simulink model "Demo_LaneKeeping_cs"  (Simulink 8.7)
settings: Solver=ode5  SolverMode=SingleTasking  StartTime=0.0  StopTime=38  FixedStep=1/20  RelTol=1e-3
model workspace (MAT data in the model file):
  mbox_table.block_array(1).src = 'built-in/Subsystem'
  mbox_table.block_array(1).dest = 'Demo_LaneKeeping_cs/Mazda_RX8_1'
  mbox_table.block_array(1).mode = 0
  mbox_table.block_array(2).src = 'simulink/Sinks/Out1'
  mbox_table.block_array(2).dest = 'Demo_LaneKeeping_cs/Mazda_RX8_1/STATE_Mazda_RX8_1'
  mbox_table.block_array(2).mode = 0
  mbox_table.block_array(3).src = 'PreScanSimulinkLibrary/State'
  mbox_table.block_array(3).dest = 'Demo_LaneKeeping_cs/STATE_Mazda_RX8_1'
  mbox_table.block_array(3).mode = 0
  mbox_table.block_array(4).src = 'PreScanSimulinkLibrary/SELF'
  mbox_table.block_array(4).dest = 'Demo_LaneKeeping_cs/SELF_Mazda_RX8_1'
  mbox_table.block_array(4).mode = 0
  mbox_table.block_array(5).src = 'simulink/Sources/In1'
  mbox_table.block_array(5).dest = 'Demo_LaneKeeping_cs/Mazda_RX8_1/SELF_Mazda_RX8_1'
  mbox_table.block_array(5).mode = 0
  mbox_table.block_array(6).src = 'PreScanSimulinkLibrary/DemuxSELF'
  mbox_table.block_array(6).dest = 'Demo_LaneKeeping_cs/Mazda_RX8_1/SELF_Demux'
  mbox_table.block_array(6).mode = 0
  mbox_table.block_array(7).src = 'PreScanSimulinkLibrary/LaneMarkerSensor'
  mbox_table.block_array(7).dest = 'Demo_LaneKeeping_cs/LaneMarkerSensor_1'
  mbox_table.block_array(7).mode = 0
  mbox_table.block_array(8).src = 'simulink/Sources/In1'
  mbox_table.block_array(8).dest = 'Demo_LaneKeeping_cs/Mazda_RX8_1/LaneMarkerSensor_1'
  mbox_table.block_array(8).mode = 0
  mbox_table.block_array(9).src = 'PreScanSimulinkLibrary/LaneMarkerSensor_Data'
  mbox_table.block_array(9).dest = 'Demo_LaneKeeping_cs/Mazda_RX8_1/LaneMarkerSensor_1_Data'
  mbox_table.block_array(9).mode = 0
  mbox_table.block_array(10).src = 'simulink/Sinks/Out1'
  mbox_table.block_array(10).dest = 'Demo_LaneKeeping_cs/Mazda_RX8_1/VISUWheels_Mazda_RX8_1'
  mbox_table.block_array(10).mode = 0
  mbox_table.block_array(11).src = 'PreScanSimulinkLibrary/VisuWheels'
  mbox_table.block_array(11).dest = 'Demo_LaneKeeping_cs/VISUWheels_Mazda_RX8_1'
  mbox_table.block_array(11).mode = 0
  mbox_table.block_array(12).src = 'PreScanSimulinkLibrary/MuxWheels'
  mbox_table.block_array(12).dest = 'Demo_LaneKeeping_cs/Mazda_RX8_1/VISUWheels_Mux'
  mbox_table.block_array(12).mode = 0
  mbox_table.block_array(13).src = 'simulink/Sinks/Out1'
  mbox_table.block_array(13).dest = 'Demo_LaneKeeping_cs/Mazda_RX8_1/VISUSteer_Mazda_RX8_1'
  mbox_table.block_array(13).mode = 0
  mbox_table.block_array(14).src = 'PreScanSimulinkLibrary/VisuSteer'
  mbox_table.block_array(14).dest = 'Demo_LaneKeeping_cs/VISUSteer_Mazda_RX8_1'
  mbox_table.block_array(14).mode = 0
  mbox_table.block_array(15).src = 'PreScanSimulinkLibrary/MuxSteer'
  mbox_table.block_array(15).dest = 'Demo_LaneKeeping_cs/Mazda_RX8_1/VISUSteer_Mux'
  mbox_table.block_array(15).mode = 0
  mbox_table.block_array(16).src = 'PreScanSimulinkLibrary/Simple_Vehicle_Dynamics'
  mbox_table.block_array(16).dest = 'Demo_LaneKeeping_cs/Mazda_RX8_1/Dynamics_Simple'
  mbox_table.block_array(16).mode = 0
  mbox_table.block_array(17).src = 'simulink/Sources/Constant'
  mbox_table.block_array(17).dest = 'Demo_LaneKeeping_cs/Mazda_RX8_1/Auto_Gear'
  mbox_table.block_array(17).mode = 0
  mbox_table.block_array(18).src = 'SimCoreLibrary/SimCoreConfiguration'
  mbox_table.block_array(18).dest = 'Demo_LaneKeeping_cs/SimCoreConfiguration'
  mbox_table.block_array(18).mode = 0
  mbox_table.block_array(19).src = 'SimCoreLibrary/Actuators'
  mbox_table.block_array(19).dest = 'Demo_LaneKeeping_cs/Actuators'
  mbox_table.block_array(19).mode = 0
  mbox_table.block_array(20).src = 'SimCoreLibrary/SetActuators'
  mbox_table.block_array(20).dest = 'Demo_LaneKeeping_cs/SetActuators'
  mbox_table.block_array(20).mode = 0
  mbox_table.block_array(21).src = 'SimCoreLibrary/GetSensors'
  mbox_table.block_array(21).dest = 'Demo_LaneKeeping_cs/GetSensors'
  mbox_table.block_array(21).mode = 0
  mbox_table.block_array(22).src = 'SimCoreLibrary/SimCoreInfo'
  mbox_table.block_array(22).dest = 'Demo_LaneKeeping_cs/SimCoreInfo'
  mbox_table.block_array(22).mode = 0
  mbox_table.block_array(23).src = 'PreScanSimulinkLibrary/Regenerate'
  mbox_table.block_array(23).dest = 'Demo_LaneKeeping_cs/Regenerate'
  mbox_table.block_array(23).mode = 0
  mbox_table.block_array(24).src = 'PreScanSimulinkLibrary/Record for Replay  '
  mbox_table.block_array(24).dest = 'Demo_LaneKeeping_cs/Record for Replay  '
  mbox_table.block_array(24).mode = 0
  mbox_table.block_array(25).src = 'PreScanSimulinkLibrary/Open Useful Blocks'
  mbox_table.block_array(25).dest = 'Demo_LaneKeeping_cs/Open Useful Blocks'
  mbox_table.block_array(25).mode = 0
  mbox_table.block_array(26).src = 'PreScanSimulinkLibrary/PreScan Options   '
  mbox_table.block_array(26).dest = 'Demo_LaneKeeping_cs/PreScan Options   '
  mbox_table.block_array(26).mode = 0
  mbox_table.block_array(27).src = 'built-in/Note'
  mbox_table.block_array(27).dest = 'Demo_LaneKeeping_cs/Version:                  '
  mbox_table.block_array(27).mode = 0
  mbox_table.block_array(28).src = 'built-in/Note'
  mbox_table.block_array(28).dest = 'Demo_LaneKeeping_cs/7.4.0'
  mbox_table.block_array(28).mode = 0
  mbox_table.block_array(29).src = 'built-in/Note'
  mbox_table.block_array(29).dest = 'Demo_LaneKeeping_cs/Author(s):                '
  mbox_table.block_array(29).mode = 0
  mbox_table.block_array(30).src = 'built-in/Note'
  mbox_table.block_array(30).dest = 'Demo_LaneKeeping_cs/A. Pastore'
  mbox_table.block_array(30).mode = 0
  mbox_table.block_array(31).src = 'built-in/Note'
  mbox_table.block_array(31).dest = 'Demo_LaneKeeping_cs/Descriptive text:      '
  mbox_table.block_array(31).mode = 0
  mbox_table.block_array(32).src = 'built-in/Note'
  mbox_table.block_array(32).dest = 'Demo_LaneKeeping_cs/Lane Keeping Assist System Demo.'
  mbox_table.block_array(32).mode = 0
  mbox_table.block_array(33).src = 'built-in/Note'
  mbox_table.block_array(33).dest = 'Demo_LaneKeeping_cs/ID
    | 
    | 1'
  mbox_table.block_array(33).mode = 0
  mbox_table.block_array(34).src = 'built-in/Note'
  mbox_table.block_array(34).dest = 'Demo_LaneKeeping_cs/OBU-Beacon ID
    | 
    | '
  mbox_table.block_array(34).mode = 0
  mbox_table.block_array(35).src = 'built-in/Note'
  mbox_table.block_array(35).dest = 'Demo_LaneKeeping_cs/TypeID
    | 
    | 1'
  mbox_table.block_array(35).mode = 0
  mbox_table.block_array(36).src = 'built-in/Note'
  mbox_table.block_array(36).dest = 'Demo_LaneKeeping_cs/TypeTag
    | 
    | Car'
  mbox_table.block_array(36).mode = 0
  mbox_table.block_array(37).src = 'built-in/Note'
  mbox_table.block_array(37).dest = 'Demo_LaneKeeping_cs/SD
    | 
    | Y'
  mbox_table.block_array(37).mode = 0
  mbox_table.block_array(38).src = 'built-in/Note'
  mbox_table.block_array(38).dest = 'Demo_LaneKeeping_cs/CD
    | 
    | N'
  mbox_table.block_array(38).mode = 0
  mbox_table.block_array(39).src = 'built-in/Note'
  mbox_table.block_array(39).dest = 'Demo_LaneKeeping_cs/Name
    | 
    | Mazda_RX8_1'
  mbox_table.block_array(39).mode = 0
  mbox_table.block_array(40).src = 'built-in/Note'
  mbox_table.block_array(40).dest = 'Demo_LaneKeeping_cs/Num ID       OBU-Beacon ID     Type ID      Type Tag             SD        CD             Name                          '
  mbox_table.block_array(40).mode = 0
  mbox_table.block_array(41).src = 'built-in/Ground'
  mbox_table.block_array(41).dest = 'Demo_LaneKeeping_cs/Mazda_RX8_1/Ground_1'
  mbox_table.block_array(41).mode = 1
  mbox_table.block_array(42).src = 'built-in/Ground'
  mbox_table.block_array(42).dest = 'Demo_LaneKeeping_cs/Mazda_RX8_1/Ground_2'
  mbox_table.block_array(42).mode = 1
  mbox_table.block_array(43).src = 'built-in/Ground'
  mbox_table.block_array(43).dest = 'Demo_LaneKeeping_cs/Mazda_RX8_1/Ground_3'
  mbox_table.block_array(43).mode = 1
  mbox_table.block_array(44).src = 'built-in/Ground'
  mbox_table.block_array(44).dest = 'Demo_LaneKeeping_cs/Mazda_RX8_1/Ground_4'
  mbox_table.block_array(44).mode = 1
  mbox_table.block_array(45).src = 'built-in/Terminator'
  mbox_table.block_array(45).dest = 'Demo_LaneKeeping_cs/Mazda_RX8_1/Terminator_1'
  mbox_table.block_array(45).mode = 1
  mbox_table.block_array(46).src = 'built-in/Terminator'
  mbox_table.block_array(46).dest = 'Demo_LaneKeeping_cs/Mazda_RX8_1/Terminator_2'
  mbox_table.block_array(46).mode = 1
  mbox_table.block_array(47).src = 'built-in/Terminator'
  mbox_table.block_array(47).dest = 'Demo_LaneKeeping_cs/Mazda_RX8_1/Terminator_3'
  mbox_table.block_array(47).mode = 1
  mbox_table.block_array(48).src = 'built-in/Terminator'
  mbox_table.block_array(48).dest = 'Demo_LaneKeeping_cs/Mazda_RX8_1/Terminator_4'
  mbox_table.block_array(48).mode = 1
  mbox_table.block_array(49).src = 'built-in/Terminator'
  mbox_table.block_array(49).dest = 'Demo_LaneKeeping_cs/Mazda_RX8_1/Terminator_5'
  mbox_table.block_array(49).mode = 1
  mbox_table.block_array(50).src = 'built-in/Terminator'
  mbox_table.block_array(50).dest = 'Demo_LaneKeeping_cs/Mazda_RX8_1/Terminator_6'
  mbox_table.block_array(50).mode = 1
  mbox_table.block_array(51).src = 'built-in/Terminator'
  mbox_table.block_array(51).dest = 'Demo_LaneKeeping_cs/Mazda_RX8_1/Terminator_7'
  mbox_table.block_array(51).mode = 1
  mbox_table.block_array(52).src = 'built-in/Terminator'
  mbox_table.block_array(52).dest = 'Demo_LaneKeeping_cs/Mazda_RX8_1/Terminator_8'
  mbox_table.block_array(52).mode = 1
  mbox_table.block_array(53).src = 'built-in/Terminator'
  mbox_table.block_array(53).dest = 'Demo_LaneKeeping_cs/Mazda_RX8_1/Terminator_9'
  mbox_table.block_array(53).mode = 1
  mbox_table.block_array(54).src = 'built-in/Terminator'
  mbox_table.block_array(54).dest = 'Demo_LaneKeeping_cs/Mazda_RX8_1/Terminator_10'
  mbox_table.block_array(54).mode = 1
  mbox_table.block_array(55).src = 'built-in/Terminator'
  mbox_table.block_array(55).dest = 'Demo_LaneKeeping_cs/Mazda_RX8_1/Terminator_11'
  mbox_table.block_array(55).mode = 1
  mbox_table.block_array(56).src = 'built-in/Terminator'
  mbox_table.block_array(56).dest = 'Demo_LaneKeeping_cs/Mazda_RX8_1/Terminator_12'
  mbox_table.block_array(56).mode = 1
  mbox_table.block_array(57).src = 'built-in/Terminator'
  mbox_table.block_array(57).dest = 'Demo_LaneKeeping_cs/Mazda_RX8_1/Terminator_13'
  mbox_table.block_array(57).mode = 1
  mbox_table.block_array(58).src = 'built-in/Ground'
  mbox_table.block_array(58).dest = 'Demo_LaneKeeping_cs/Mazda_RX8_1/Ground_5'
  mbox_table.block_array(58).mode = 1
  mbox_table.block_array(59).src = 'built-in/Ground'
  mbox_table.block_array(59).dest = 'Demo_LaneKeeping_cs/Mazda_RX8_1/Ground_6'
  mbox_table.block_array(59).mode = 1
  mbox_table.block_array(60).src = 'built-in/Ground'
  mbox_table.block_array(60).dest = 'Demo_LaneKeeping_cs/Mazda_RX8_1/Ground_7'
  mbox_table.block_array(60).mode = 1
  mbox_table.block_array(61).src = 'built-in/Ground'
  mbox_table.block_array(61).dest = 'Demo_LaneKeeping_cs/Mazda_RX8_1/Ground_8'
  mbox_table.block_array(61).mode = 1
  mbox_table.block_array(62).src = 'built-in/Ground'
  mbox_table.block_array(62).dest = 'Demo_LaneKeeping_cs/Mazda_RX8_1/Ground_9'
  mbox_table.block_array(62).mode = 1
  mbox_table.block_index : java.util.Hashtable (value not decoded)
  mbox_table.line_array(1).sys = 'Demo_LaneKeeping_cs'
  mbox_table.line_array(1).line_id = 'L1'
  mbox_table.line_array(1).iport = 'STATE_Mazda_RX8_1/1'
  mbox_table.line_array(1).oport = 'Mazda_RX8_1/1'
  mbox_table.line_array(1).mode = 0
  mbox_table.line_array(2).sys = 'Demo_LaneKeeping_cs'
  mbox_table.line_array(2).line_id = 'L2'
  mbox_table.line_array(2).iport = 'Mazda_RX8_1/1'
  mbox_table.line_array(2).oport = 'SELF_Mazda_RX8_1/1'
  mbox_table.line_array(2).mode = 0
  mbox_table.line_array(3).sys = 'Demo_LaneKeeping_cs/Mazda_RX8_1'
  mbox_table.line_array(3).line_id = 'L3'
  mbox_table.line_array(3).iport = 'SELF_Demux/1'
  mbox_table.line_array(3).oport = 'SELF_Mazda_RX8_1/1'
  mbox_table.line_array(3).mode = 0
  mbox_table.line_array(4).sys = 'Demo_LaneKeeping_cs/Mazda_RX8_1'
  mbox_table.line_array(4).line_id = 'L4'
  mbox_table.line_array(4).iport = 'LaneMarkerSensor_1_Data/1'
  mbox_table.line_array(4).oport = 'LaneMarkerSensor_1/1'
  mbox_table.line_array(4).mode = 0
  mbox_table.line_array(5).sys = 'Demo_LaneKeeping_cs'
  mbox_table.line_array(5).line_id = 'L5'
  mbox_table.line_array(5).iport = 'Mazda_RX8_1/2'
  mbox_table.line_array(5).oport = 'LaneMarkerSensor_1/1'
  mbox_table.line_array(5).mode = 0
  mbox_table.line_array(6).sys = 'Demo_LaneKeeping_cs/Mazda_RX8_1'
  mbox_table.line_array(6).line_id = 'L6'
  mbox_table.line_array(6).iport = 'VISUWheels_Mazda_RX8_1/1'
  mbox_table.line_array(6).oport = 'VISUWheels_Mux/1'
  mbox_table.line_array(6).mode = 0
  mbox_table.line_array(7).sys = 'Demo_LaneKeeping_cs'
  mbox_table.line_array(7).line_id = 'L7'
  mbox_table.line_array(7).iport = 'VISUWheels_Mazda_RX8_1/1'
  mbox_table.line_array(7).oport = 'Mazda_RX8_1/2'
  mbox_table.line_array(7).mode = 0
  mbox_table.line_array(8).sys = 'Demo_LaneKeeping_cs/Mazda_RX8_1'
  mbox_table.line_array(8).line_id = 'L8'
  mbox_table.line_array(8).iport = 'VISUSteer_Mazda_RX8_1/1'
  mbox_table.line_array(8).oport = 'VISUSteer_Mux/1'
  mbox_table.line_array(8).mode = 0
  mbox_table.line_array(9).sys = 'Demo_LaneKeeping_cs'
  mbox_table.line_array(9).line_id = 'L9'
  mbox_table.line_array(9).iport = 'VISUSteer_Mazda_RX8_1/1'
  mbox_table.line_array(9).oport = 'Mazda_RX8_1/3'
  mbox_table.line_array(9).mode = 0
  mbox_table.line_array(10).sys = 'Demo_LaneKeeping_cs/Mazda_RX8_1'
  mbox_table.line_array(10).line_id = 'L10'
  mbox_table.line_array(10).iport = 'VISUWheels_Mux/3'
  mbox_table.line_array(10).oport = 'Dynamics_Simple/2'
  mbox_table.line_array(10).mode = 0
  mbox_table.line_array(11).sys = 'Demo_LaneKeeping_cs/Mazda_RX8_1'
  mbox_table.line_array(11).line_id = 'L11'
  mbox_table.line_array(11).iport = 'Dynamics_Simple/6'
  mbox_table.line_array(11).oport = 'Auto_Gear/1'
  mbox_table.line_array(11).mode = 0
  mbox_table.line_array(12).sys = 'Demo_LaneKeeping_cs/Mazda_RX8_1'
  mbox_table.line_array(12).line_id = 'L12'
  mbox_table.line_array(12).iport = 'STATE_Mazda_RX8_1/1'
  mbox_table.line_array(12).oport = 'Dynamics_Simple/1'
  mbox_table.line_array(12).mode = 0
  mbox_table.line_array(13).sys = 'Demo_LaneKeeping_cs/Mazda_RX8_1'
  mbox_table.line_array(13).line_id = 'l1'
  mbox_table.line_array(13).iport = 'Dynamics_Simple/3'
  mbox_table.line_array(13).oport = 'Ground_1/1'
  mbox_table.line_array(13).mode = 1
  mbox_table.line_array(14).sys = 'Demo_LaneKeeping_cs/Mazda_RX8_1'
  mbox_table.line_array(14).line_id = 'l2'
  mbox_table.line_array(14).iport = 'Dynamics_Simple/4'
  mbox_table.line_array(14).oport = 'Ground_2/1'
  mbox_table.line_array(14).mode = 1
  mbox_table.line_array(15).sys = 'Demo_LaneKeeping_cs/Mazda_RX8_1'
  mbox_table.line_array(15).line_id = 'l3'
  mbox_table.line_array(15).iport = 'Dynamics_Simple/5'
  mbox_table.line_array(15).oport = 'Ground_3/1'
  mbox_table.line_array(15).mode = 1
  mbox_table.line_array(16).sys = 'Demo_LaneKeeping_cs/Mazda_RX8_1'
  mbox_table.line_array(16).line_id = 'l4'
  mbox_table.line_array(16).iport = 'Dynamics_Simple/7'
  mbox_table.line_array(16).oport = 'Ground_4/1'
  mbox_table.line_array(16).mode = 1
  mbox_table.line_array(17).sys = 'Demo_LaneKeeping_cs/Mazda_RX8_1'
  mbox_table.line_array(17).line_id = 'l5'
  mbox_table.line_array(17).iport = 'Terminator_1/1'
  mbox_table.line_array(17).oport = 'Dynamics_Simple/3'
  mbox_table.line_array(17).mode = 1
  mbox_table.line_array(18).sys = 'Demo_LaneKeeping_cs/Mazda_RX8_1'
  mbox_table.line_array(18).line_id = 'l6'
  mbox_table.line_array(18).iport = 'Terminator_2/1'
  mbox_table.line_array(18).oport = 'SELF_Demux/1'
  mbox_table.line_array(18).mode = 1
  mbox_table.line_array(19).sys = 'Demo_LaneKeeping_cs/Mazda_RX8_1'
  mbox_table.line_array(19).line_id = 'l7'
  mbox_table.line_array(19).iport = 'Terminator_3/1'
  mbox_table.line_array(19).oport = 'SELF_Demux/2'
  mbox_table.line_array(19).mode = 1
  mbox_table.line_array(20).sys = 'Demo_LaneKeeping_cs/Mazda_RX8_1'
  mbox_table.line_array(20).line_id = 'l8'
  mbox_table.line_array(20).iport = 'Terminator_4/1'
  mbox_table.line_array(20).oport = 'SELF_Demux/3'
  mbox_table.line_array(20).mode = 1
  mbox_table.line_array(21).sys = 'Demo_LaneKeeping_cs/Mazda_RX8_1'
  mbox_table.line_array(21).line_id = 'l9'
  mbox_table.line_array(21).iport = 'Terminator_5/1'
  mbox_table.line_array(21).oport = 'SELF_Demux/4'
  mbox_table.line_array(21).mode = 1
  mbox_table.line_array(22).sys = 'Demo_LaneKeeping_cs/Mazda_RX8_1'
  mbox_table.line_array(22).line_id = 'l10'
  mbox_table.line_array(22).iport = 'Terminator_6/1'
  mbox_table.line_array(22).oport = 'SELF_Demux/5'
  mbox_table.line_array(22).mode = 1
  mbox_table.line_array(23).sys = 'Demo_LaneKeeping_cs/Mazda_RX8_1'
  mbox_table.line_array(23).line_id = 'l11'
  mbox_table.line_array(23).iport = 'Terminator_7/1'
  mbox_table.line_array(23).oport = 'SELF_Demux/6'
  mbox_table.line_array(23).mode = 1
  mbox_table.line_array(24).sys = 'Demo_LaneKeeping_cs/Mazda_RX8_1'
  mbox_table.line_array(24).line_id = 'l12'
  mbox_table.line_array(24).iport = 'Terminator_8/1'
  mbox_table.line_array(24).oport = 'SELF_Demux/7'
  mbox_table.line_array(24).mode = 1
  mbox_table.line_array(25).sys = 'Demo_LaneKeeping_cs/Mazda_RX8_1'
  mbox_table.line_array(25).line_id = 'l13'
  mbox_table.line_array(25).iport = 'Terminator_9/1'
  mbox_table.line_array(25).oport = 'SELF_Demux/8'
  mbox_table.line_array(25).mode = 1
  mbox_table.line_array(26).sys = 'Demo_LaneKeeping_cs/Mazda_RX8_1'
  mbox_table.line_array(26).line_id = 'l14'
  mbox_table.line_array(26).iport = 'Terminator_10/1'
  mbox_table.line_array(26).oport = 'SELF_Demux/9'
  mbox_table.line_array(26).mode = 1
  mbox_table.line_array(27).sys = 'Demo_LaneKeeping_cs/Mazda_RX8_1'
  mbox_table.line_array(27).line_id = 'l15'
  mbox_table.line_array(27).iport = 'Terminator_11/1'
  mbox_table.line_array(27).oport = 'SELF_Demux/10'
  mbox_table.line_array(27).mode = 1
  mbox_table.line_array(28).sys = 'Demo_LaneKeeping_cs/Mazda_RX8_1'
  mbox_table.line_array(28).line_id = 'l16'
  mbox_table.line_array(28).iport = 'Terminator_12/1'
  mbox_table.line_array(28).oport = 'SELF_Demux/11'
  mbox_table.line_array(28).mode = 1
  mbox_table.line_array(29).sys = 'Demo_LaneKeeping_cs/Mazda_RX8_1'
  mbox_table.line_array(29).line_id = 'l17'
  mbox_table.line_array(29).iport = 'Terminator_13/1'
  mbox_table.line_array(29).oport = 'SELF_Demux/12'
  mbox_table.line_array(29).mode = 1
  mbox_table.line_array(30).sys = 'Demo_LaneKeeping_cs/Mazda_RX8_1'
  mbox_table.line_array(30).line_id = 'l18'
  mbox_table.line_array(30).iport = 'VISUWheels_Mux/2'
  mbox_table.line_array(30).oport = 'Ground_5/1'
  mbox_table.line_array(30).mode = 1
  mbox_table.line_array(31).sys = 'Demo_LaneKeeping_cs/Mazda_RX8_1'
  mbox_table.line_array(31).line_id = 'l19'
  mbox_table.line_array(31).iport = 'VISUWheels_Mux/4'
  mbox_table.line_array(31).oport = 'Ground_6/1'
  mbox_table.line_array(31).mode = 1
  mbox_table.line_array(32).sys = 'Demo_LaneKeeping_cs/Mazda_RX8_1'
  mbox_table.line_array(32).line_id = 'l20'
  mbox_table.line_array(32).iport = 'VISUWheels_Mux/5'
  mbox_table.line_array(32).oport = 'Ground_7/1'
  mbox_table.line_array(32).mode = 1
  mbox_table.line_array(33).sys = 'Demo_LaneKeeping_cs/Mazda_RX8_1'
  mbox_table.line_array(33).line_id = 'l21'
  mbox_table.line_array(33).iport = 'VISUWheels_Mux/6'
  mbox_table.line_array(33).oport = 'Ground_8/1'
  mbox_table.line_array(33).mode = 1
  mbox_table.line_array(34).sys = 'Demo_LaneKeeping_cs/Mazda_RX8_1'
  mbox_table.line_array(34).line_id = 'l22'
  mbox_table.line_array(34).iport = 'VISUWheels_Mux/7'
  mbox_table.line_array(34).oport = 'Ground_9/1'
  mbox_table.line_array(34).mode = 1
  mbox_table.line_index : java.util.Hashtable (value not decoded)
  mbox_table.next_linenr = 13
  mbox_table.next_termlinenr = 23
  model_closed = 0
  sim_status = 0
PreLoadFcn:
  | check_NUTS_defined;
  | 
  | assignin('base',['model_closed_' bdroot],false);
InitFcn:
  | PreScanExperimentInitFcn(bdroot)
StopFcn:
  | PreScanExperimentStopFcn(bdroot)
undefined symbols (not defined in the file or in its folder): DiscIntNeverNeededParam, x_ini_VRML, y_ini_VRML, z_ini_VRML
libraries: simulink x18, simulink_extras x4, PreScanSimulinkLibrary x2, PreScanUsefulBlocks x1
(part 1 of 3)
CloseFcn:
  | evalin('base',['clear model_closed_' bdroot]);
settings Model: Creator=PRESCAN  LastModifiedBy=agrawal
settings DataIOCC: InspectSignalLogs=on  LoggingToFile=on  LoggingFileName=out-Lane.mat
settings OptimizationCC: ExpressionDepthLimit=2147483647  InitFltsAndDblsToZero=on
settings DebuggingCC: SaveWithParameterizedLinksMsg=none  SignalResolutionControl=TryResolveAllWithWarning  SolverPrmCheckMsg=warning  MultiTaskDSMMsg=warning  MultiTaskCondExecSysMsg=none  FcnCallInpInsideContextMsg=UseLocalSettings  StateNameClashWarn=warning
settings GRTTargetCC: TargetFcnLib=ansi_tfl_tmw.mat  CombineOutputUpdateFcns=off  GRTInterface=on

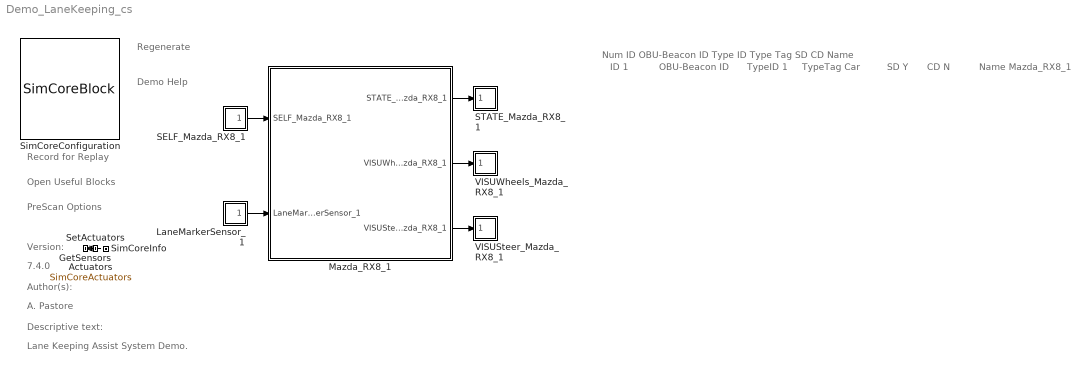
== system Demo_LaneKeeping_cs ==
  note: Demo Help
  note: Regenerate
  note: Record for Replay
  note: Open Useful Blocks
  note: PreScan Options
  note: Version:
  note: 7.4.0
  note: Author(s):
  note: A. Pastore
  note: Descriptive text:
  note: Lane Keeping Assist System Demo.
  note: ID
      |
      | 1
  note: OBU-Beacon ID
  note: TypeID
      |
      | 1
  note: TypeTag
      |
      | Car
  note: SD
      |
      | Y
  note: CD
      |
      | N
  note: Name
      |
      | Mazda_RX8_1
  note: Num ID OBU-Beacon ID Type ID Type Tag SD CD Name
  Actuators : DataStoreMemory  Tag=Actuators  DataStoreName=SimCoreActuators  InitialValue=zeros(51,1)  ShowAdditionalParam=off
      settings: DeleteFcn=PreScanBlockDeleteFcn;
  GetSensors : Subsystem  Tag=GetSensors  Priority=2  mask(PreScan Simulation Core Block){NrOfSensors=8, TimeStep=1/20}
      mask prompts: NrOfSensors "Number of sensor values"; TimeStep "Timestep [s]"
      mask help:
      | Please do not remove this block from the PreScan compilation sheet,
      | as it contains essential configuration parameters for a PreScan simulation.
      settings: DeleteFcn=PreScanBlockDeleteFcn;
  LaneMarkerSensor_1 : Subsystem  Tag=LaneMarkerSensor  Priority=3  mask(PreScan Source Block: Lane Marker Sensor){}
      mask help: The Lane Marker Sensor provides information relating the sensor to the lane markers on the road.
      settings: DeleteFcn=PreScanBlockDeleteFcn;
      mask Help: eval('openHelp(457)')
      mask Display: image(imread('LaneMarkerSensorSL.png'))
  Mazda_RX8_1 : Subsystem  Tag=WorldObjectSubSystem  InitFcn=UniqueId = '98';
      mask Display: image(imread('Mazda_RX8.jpg'));color('white');text(0,0,' ID=1\n')
  SELF_Mazda_RX8_1 : Subsystem  Tag=SELF  Priority=3  mask(PreScan Source Block: SELF){PortName=SELF_Mazda_RX8_1, PortIndex=0, PortWidth=8, TimeStep=1/20}
      mask prompts: PortName "Auto-Assigned: Port Name [-]"; PortIndex "Auto-Assigned: Port Index [-]"; PortWidth "Auto-Assigned: Port Dimensions"; TimeStep "Auto-Assigned: Upload Period [s]"
      mask help:
      | The SELF port shows (state) information of the actor itself. The outputs are position in the experiment's axis system and the GPS coordinates, and the object's absolute velocity and compass heading.
      |
      | For more information, please click Help.
      settings: DeleteFcn=PreScanBlockDeleteFcn;
      mask Help: eval('openHelp(462)')
      mask Display: image(imread('GPS.png'))
  STATE_Mazda_RX8_1 : Subsystem  Tag=State  Priority=0  mask(PreScan Sink Block: State){x0=-23.396406173706055, y0=-52.391075134277344, z0=0.50999999046325684, Roll0=0, Pitch0=0, Yaw0=90, TimeStep=1/20}
      mask prompts: x0 "Ini x-position VEHICLE wrt GLOBAL axis system [m]"; y0 "Ini y-position VEHICLE wrt GLOBAL axis system [m]"; z0 "Ini z-position VEHICLE wrt GLOBAL axis system [m]"; Roll0 "Ini roll-angle BODY wrt VEHICLE axis system [deg]"; Pitch0 "Ini pitch-angle BODY wrt VEHICLE axis system [deg]"; Yaw0 "Ini yaw-angle VEHICLE wrt GLOBAL axis system [deg]"; TimeStep "Time Step [s]"
      mask help:
      | The Actor State contains a vector signal of size (9x1), containing the following signals:
      |
      | -  Position                  (x,y,z)                                     [m]
      | -  Velocity                  (vx,vy,vz)                               [m/s]
      | -  Angles                    (Roll, Pitch, Yaw)                   [rad]
      |
      | The Actor state is defined in the global axis system.
      | The state is superponed on the Initial position defined in the GUI.
      |
      | For more information, please click Help.
      settings: DeleteFcn=PreScanBlockDeleteFcn;
      mask Help: eval('openHelp(222)')
      mask Display: image(imread('State.png'))
  SetActuators : Subsystem  Tag=SetActuators  Priority=1  mask(PreScan Simulation Core Block){TimeStep=1/20, NrOfActuators=51}
      mask prompts: TimeStep "Timestep [s]"; NrOfActuators "Number of actuator values"
      mask help:
      | Please do not remove this block from the PreScan compilation sheet,
      | as it contains essential configuration parameters for a PreScan simulation.
      settings: DeleteFcn=PreScanBlockDeleteFcn;
  SimCoreConfiguration : M-S-Function  Tag=SimCoreConfiguration  Description=E6DFEB53D90BD3519F737E615FC0CC357B96F9EDC882605C43623E3CE783100B  FunctionName=SimCoreBlock  Parameters=ExperimentXML PortsXML SimulationCore HostName CheckStart EnableLog RfR EnableGPUAccel ShowComputationTime  mask(PreScan Simulation Core Configurator){SimulationCore=NUTS, HostName=0, CheckStart=0, prescanversion='7.4.0', EnableLog=off, RfR=0, EnableGPUAccel=off, ShowComputationTime=off}
      mask prompts: SimulationCore "Simulation Core"; HostName "Simulation Host"; CheckStart "Show START Dialog"; prescanversion "PreScan Version"; EnableLog "Create TA Log"; RfR "Record for Replay"; EnableGPUAccel "Enable GPU Acceleration"; ShowComputationTime "Show ComputationTime Scope"
      mask help:
      | Please do not remove this block from the PreScan compilation sheet,
      | as it contains essential configuration parameter for a PreScan simulation.
      mask init:
      | model = bdroot;
      | ExperimentXML = [model(1:end-3) '.pex'];
      | PortsXML = [model '_ports.pcd'];
      settings: DeleteFcn=PreScanBlockDeleteFcn;  ModelCloseFcn=assignin('base',['model_closed_' bdroot],true);
      mask Help: eval('openHelp(812)')
      mask Display: image(imread('prescanlogo.ico'))
  SimCoreInfo : Subsystem  Tag=SimCoreInfo
  VISUSteer_Mazda_RX8_1 : Subsystem  Tag=VisuSteer  Priority=0  mask(PreScan Sink Block: VisuSteer){}
      mask help:
      | The VisuSteer block provides a way to adapt the orientation of the steering column and steering wheel of a vehicle.
      |
      | For more information, please click Help.
      settings: DeleteFcn=PreScanBlockDeleteFcn;
      mask Help: eval('openHelp(223)')
      mask Display: image(imread('steeringwheel.png'))
  VISUWheels_Mazda_RX8_1 : Subsystem  Tag=VisuWheels  Priority=0  mask(PreScan Sink Block: VisuWheels){}
      mask help:
      | The VisuWheels block provides a way to animate the wheels of a vehicle, with steering, rotation (because of velocity) and z-displacement.
      |
      | For more information, please click Help.
      settings: DeleteFcn=PreScanBlockDeleteFcn;
      mask Help: eval('openHelp(223)')
      mask Display: image(imread('wheel.png'))
  wires:
  SetActuators/1(dummy) -> GetSensors/1(dummy)
  Mazda_RX8_1/1(STATE_Mazda_RX8_1) -> STATE_Mazda_RX8_1/1(State)
  SELF_Mazda_RX8_1/1(U) -> Mazda_RX8_1/1(SELF_Mazda_RX8_1)
  LaneMarkerSensor_1/1(U) -> Mazda_RX8_1/2(LaneMarkerSensor_1)
  Mazda_RX8_1/2(VISUWheels_Mazda_RX8_1) -> VISUWheels_Mazda_RX8_1/1(Wheels)
  Mazda_RX8_1/3(VISUSteer_Mazda_RX8_1) -> VISUSteer_Mazda_RX8_1/1(Steer)

== system Demo_LaneKeeping_cs/GetSensors ==
  dummy : Inport
  GetSensors : M-S-Function  FunctionName=GetSensorsBlock  Parameters=TimeStep NrOfSensors
  tag scope: SimCoreSensors=global
  wires:
  GetSensors/1 -> [SimCoreSensors]
  dummy/1 -> GetSensors/1

== system Demo_LaneKeeping_cs/LaneMarkerSensor_1 ==
  Demux : Demux  Outputs=[1 -1]
  Terminator : Terminator
  U : Outport
  wires:
  Demux/2 -> Terminator/1
  Demux/1 -> U/1
  [SimCoreSensors] -> Demux/1

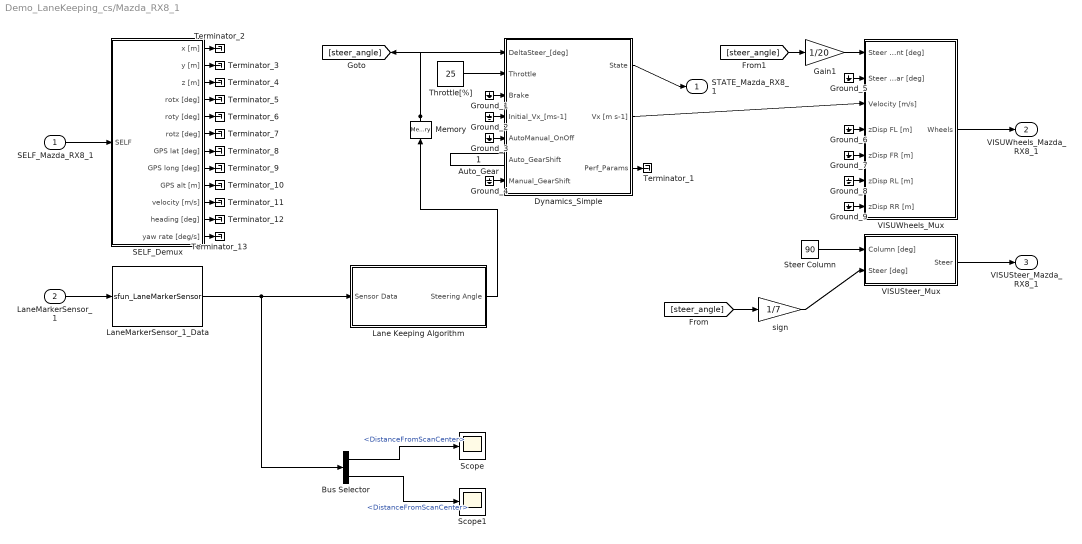
== system Demo_LaneKeeping_cs/Mazda_RX8_1 ==
  SELF_Mazda_RX8_1 : Inport  Tag=SELFInport
  LaneMarkerSensor_1 : Inport  Tag=LaneMarkerSensorInport  Port=2  SampleTime=1/20
  Auto_Gear : Constant  Tag=AutoGear
  Bus Selector : BusSelector  OutputSignals=ScanAtDistance1.LeftLaneIntersection1.DistanceFromScanCenter,ScanAtDistance1.RightLaneIntersection1.DistanceFromScanCenter
  Dynamics_Simple : Subsystem  Tag=Simple_Vehicle_Dynamics  mask(PreScan Block: Simple Dynamics){Migrate=on, TimeStep=1/20, ComputationMode=Continuous_Time}
      mask prompts: Migrate "Migrate. During migration this block will be replaced by a newer one."; TimeStep "Auto assigned: Time Step [s]"; ComputationMode "Computation mode:"
      mask help:
      | The Simple Dynamics Model is selected in the GUI to simulate vehicle dynamics behavior.
      |
      | The Simple Dynamics Model is completely open to the user. The parameters of this model can be set in the Simple Dynamics dialog in the GUI.
      |
      | For more information, please click Help.
      mask init:
      | p = SimpleDyn_pars;
      settings: DeleteFcn=PreScanBlockDeleteFcn;
      mask Help: eval('openHelp(220)')
      mask Display:
      | image(imread('SimpleDyn.png'))
      | port_label('input', 1, '{\delta}_S_t_ _e_e_r [deg]','texmode','on')
      | port_label('input', 2, 'Throttle [%]')
      | port_label('input', 3, 'Brake Pres [bar]')
      | port_label('input', 4, 'V_0 [ms-1]','texmode','on')
      | port_label('input', 5, 'Auto=[0]/Manual=[1]')
      | port_label('input', 6, 'Auto_GearShift')
      | port_label('input', 7, 'Manual_GearShift')
      | port_label('output', 1, 'State')
      | port_label('output', 2, 'Vx [ms-1]')
      | port_label('output', 3, 'Perf Params')
  Gain1 : Gain  Gain=1/20
  Ground_{1..9} (9 alike) : Ground
  Lane Keeping Algorithm : Subsystem
  LaneMarkerSensor_1_Data : S-Function  Tag=LaneMarkerSensor_Data  LoadFcn=load('LaneMarkerSensorBusses.mat');  FunctionName=sfun_LaneMarkerSensor  Parameters=[VerticalResolution HorizontalResolution] FrameRate SensorName OutputReferenceImage SharedMemTag SharedMemDataTag  SFunctionDeploymentMode=off  EnableBusSupport=on  mask{HorizontalResolution=320, VerticalResolution=240, FrameRate=20, SensorName=LaneMarkerSensor_1, OutputReferenceImage=off, SharedMemTag=LaneMarkerSensor_1_monoBeam_viewer_RGB, SharedMemDataTag=LaneMarkerSensor_1_monoBeam_viewer_LMS_Data}
      mask prompts: HorizontalResolution "User Specified: Horizontal Resolution [pixels]"; VerticalResolution "User Specified: Vertical Resolution [pixels]"; FrameRate "User Specified: Frame Rate [Hz]"; SensorName "User Specified: Lane Marker Sensor Name"; OutputReferenceImage "User Specified: Output Reference Image"; SharedMemTag "Tag for shared memory for lane marker img"; SharedMemDataTag "Tag for shared memory data"
      mask init:
      | DataPort = 1;
      | if OutputReferenceImage==1
      |     Rport = 2;
      |     Gport = 3;
      |     Bport = 4;
      |     RportName = 'Ref. Image R';
      |     GportName = 'Ref. Image G';
      |     BportName = 'Ref. Image B';
      | else
      |     Rport = 1;
      |     Gport = 1;
      |     Bport = 1;
      |     RportName = '';
      |     GportName = '';
      |     BportName = '';
      | end
      settings: DeleteFcn=PreScanBlockDeleteFcn;
      mask Display:
      | port_label('output',DataPort,'Detection Data')
      | port_label('output',Rport,RportName)
      | port_label('output',Gport,GportName)
      | port_label('output',Bport,BportName)
  Memory : Memory
  SELF_Demux : Subsystem  Tag=DemuxSELF  mask(PreScan Demux Block:){}
      settings: DeleteFcn=PreScanBlockDeleteFcn;
      mask Display:
      | port_label('output',1,'x [m]')
      | port_label('output',2,'y [m]')
      | port_label('output',3,'z [m]','texmode','on')
      | port_label('output',4,'Rotx [deg]','texmode','on')
      | port_label('output',5,'Roty [deg]','texmode','on')
      | port_label('output',6,'Rotz [deg]','texmode','on')
      | port_label('output',7,'GPS lat [deg]','texmode','on')
      | port_label('output',8,'GPS long [deg]','texmode','on')
      | port_label('output',9,'GPS alt [m]','texmode','on')
      | port_label('output',10,'Velocity [m/s]')
      | port_label('output',11,'Heading [deg]')
      | port_label('output',12,'Yaw rate [deg/s]')
  Scope : Scope
  Scope1 : Scope
  Steer Column : Constant  Value=90
  Terminator_{1..13} (13 alike) : Terminator
  Throttle[%] : Constant  Value=25
  VISUSteer_Mux : Subsystem  Tag=MuxSteer  mask(PreScan Mux Block:){}
      settings: DeleteFcn=PreScanBlockDeleteFcn;
  VISUWheels_Mux : Subsystem  Tag=MuxWheels  mask(PreScan Mux Block:){TimeStep=1/20}
      mask prompts: TimeStep "Auto Assigned: Time Step [s]"
      settings: DeleteFcn=PreScanBlockDeleteFcn;
  sign : Gain  Gain=1/7
  STATE_Mazda_RX8_1 : Outport  Tag=StateOutport
  VISUWheels_Mazda_RX8_1 : Outport  Tag=VisuWheelsOutport  Port=2  SampleTime=1/20
  VISUSteer_Mazda_RX8_1 : Outport  Tag=VisuSteerOutport  Port=3  SampleTime=1/20
  wires:
  Lane Keeping Algorithm/1(Steering Angle) -> Memory/1
  [steer_angle] -> sign/1
  [steer_angle] -> Gain1/1
  Memory/1 -> [steer_angle], Dynamics_Simple/1(DeltaSteer_[deg])
  sign/1 -> VISUSteer_Mux/2(Steer [deg])
  LaneMarkerSensor_1_Data/1 -> Bus Selector/1, Lane Keeping Algorithm/1(Sensor Data)
  Throttle[%]/1 -> Dynamics_Simple/2(Throttle)
  Gain1/1 -> VISUWheels_Mux/1(Steer Angle Front [deg])
  Steer Column/1 -> VISUSteer_Mux/1(Column [deg])
  Bus Selector/1 -> Scope/1  "<DistanceFromScanCenter>"
  Bus Selector/2 -> Scope1/1  "<DistanceFromScanCenter>"
  SELF_Mazda_RX8_1/1 -> SELF_Demux/1(SELF)
  LaneMarkerSensor_1/1 -> LaneMarkerSensor_1_Data/1
  VISUWheels_Mux/1(Wheels) -> VISUWheels_Mazda_RX8_1/1
  VISUSteer_Mux/1(Steer) -> VISUSteer_Mazda_RX8_1/1
  Dynamics_Simple/2(Vx [m s-1]) -> VISUWheels_Mux/3(Velocity [m/s])
  Auto_Gear/1 -> Dynamics_Simple/6(Auto_GearShift)
  Dynamics_Simple/1(State) -> STATE_Mazda_RX8_1/1
  Ground_1/1 -> Dynamics_Simple/3(Brake)
  Ground_2/1 -> Dynamics_Simple/4(Initial_Vx_[ms-1])
  Ground_3/1 -> Dynamics_Simple/5(AutoManual_OnOff)
  Ground_4/1 -> Dynamics_Simple/7(Manual_GearShift)
  Dynamics_Simple/3(Perf_Params) -> Terminator_1/1
  SELF_Demux/1(x [m]) -> Terminator_2/1
  SELF_Demux/2(y [m]) -> Terminator_3/1
  SELF_Demux/3(z [m]) -> Terminator_4/1
  SELF_Demux/4(rotx [deg]) -> Terminator_5/1
  SELF_Demux/5(roty [deg]) -> Terminator_6/1
  SELF_Demux/6(rotz [deg]) -> Terminator_7/1
  SELF_Demux/7(GPS lat [deg]) -> Terminator_8/1
  SELF_Demux/8(GPS long [deg]) -> Terminator_9/1
  SELF_Demux/9(GPS alt [m]) -> Terminator_10/1
  SELF_Demux/10(velocity [m/s]) -> Terminator_11/1
  SELF_Demux/11(heading [deg]) -> Terminator_12/1
  SELF_Demux/12(yaw rate [deg/s]) -> Terminator_13/1
  Ground_5/1 -> VISUWheels_Mux/2(Steer Angle Rear [deg])
  Ground_6/1 -> VISUWheels_Mux/4(zDisp FL [m])
  Ground_7/1 -> VISUWheels_Mux/5(zDisp FR [m])
  Ground_8/1 -> VISUWheels_Mux/6(zDisp RL [m])
  Ground_9/1 -> VISUWheels_Mux/7(zDisp RR [m])

== system Demo_LaneKeeping_cs/SELF_Mazda_RX8_1 ==
  Selector : Selector  IndexMode=Zero-based  IndexOptions=Starting index (dialog)  Indices=PortIndex  OutputSizes=PortWidth(1)
  U : Outport
  wires:
  Selector/1 -> U/1
  [SimCoreSensors] -> Selector/1

== system Demo_LaneKeeping_cs/STATE_Mazda_RX8_1 ==
  State : Inport  SampleTime=TimeStep
  Acceleration : Subsystem  mask(ToSensorWorld){PortName=Acceleration_Mazda_RX8_1, PortIndex=6, PortWidth=3, TimeStep=1/20}
      mask prompts: PortName "Port Name [-]"; PortIndex "Index [-]"; PortWidth "Port Dimensions [-]"; TimeStep "Upload Period [s]"
      mask help: Sends signal(s) from Simulink to the Sensor World
      mask Help:
      | Sends signal(s) from Simulink to the Sensor World.
      | 
      | - Port Name [-]: specifies the name of the output terminal of the Simulink block.
      | - Index [-]: specifies the start position in the output vector sent to the Sensor World
      | - Port dimensions [-]: specifies the width (number of scalars) of the output port
      | - Upload period [s]: specifies the upload period (in seconds) of the port.
      mask Display: port_label('input', 1, PortName)
  Demux : Demux  Outputs=5
  Position : Subsystem  mask(ToSensorWorld){PortName=Position_Mazda_RX8_1, PortIndex=0, PortWidth=3, TimeStep=1/20}
      mask prompts: PortName "Port Name [-]"; PortIndex "Index [-]"; PortWidth "Port Dimensions [-]"; TimeStep "Upload Period [s]"
      mask help: Sends signal(s) from Simulink to the Sensor World
      mask Help:
      | Sends signal(s) from Simulink to the Sensor World.
      | 
      | - Port Name [-]: specifies the name of the output terminal of the Simulink block.
      | - Index [-]: specifies the start position in the output vector sent to the Sensor World
      | - Port dimensions [-]: specifies the width (number of scalars) of the output port
      | - Upload period [s]: specifies the upload period (in seconds) of the port.
      mask Display: port_label('input', 1, PortName)
  RPY : Subsystem  mask(ToSensorWorld){PortName=RPY_Mazda_RX8_1, PortIndex=9, PortWidth=3, TimeStep=1/20}
      mask prompts: PortName "Port Name [-]"; PortIndex "Index [-]"; PortWidth "Port Dimensions [-]"; TimeStep "Upload Period [s]"
      mask help: Sends signal(s) from Simulink to the Sensor World
      mask Help:
      | Sends signal(s) from Simulink to the Sensor World.
      | 
      | - Port Name [-]: specifies the name of the output terminal of the Simulink block.
      | - Index [-]: specifies the start position in the output vector sent to the Sensor World
      | - Port dimensions [-]: specifies the width (number of scalars) of the output port
      | - Upload period [s]: specifies the upload period (in seconds) of the port.
      mask Display: port_label('input', 1, PortName)
  Velocity : Subsystem  mask(ToSensorWorld){PortName=Velocity_Mazda_RX8_1, PortIndex=3, PortWidth=3, TimeStep=1/20}
      mask prompts: PortName "Port Name [-]"; PortIndex "Index [-]"; PortWidth "Port Dimensions [-]"; TimeStep "Upload Period [s]"
      mask help: Sends signal(s) from Simulink to the Sensor World
      mask Help:
      | Sends signal(s) from Simulink to the Sensor World.
      | 
      | - Port Name [-]: specifies the name of the output terminal of the Simulink block.
      | - Index [-]: specifies the start position in the output vector sent to the Sensor World
      | - Port dimensions [-]: specifies the width (number of scalars) of the output port
      | - Upload period [s]: specifies the upload period (in seconds) of the port.
      mask Display: port_label('input', 1, PortName)
  iniBODYAngles wrtVEH [rad] : Constant  Value=[Roll0 Pitch0 0]  SampleTime=TimeStep
  iniVEHAngles wrtGLOB [rad] : Constant  Value=[0 0 Yaw0]  SampleTime=TimeStep
  iniVEHposition wrtGLOB [m] : Constant  Value=[x0 y0 z0]  SampleTime=TimeStep
  state2FullState : PreScanSimulinkLibrary/state2FullState  SystemSampleTime=-1
  velRPY : Subsystem  mask(ToSensorWorld){PortName=velRPY_Mazda_RX8_1, PortIndex=12, PortWidth=3, TimeStep=1/20}
      mask prompts: PortName "Port Name [-]"; PortIndex "Index [-]"; PortWidth "Port Dimensions [-]"; TimeStep "Upload Period [s]"
      mask help: Sends signal(s) from Simulink to the Sensor World
      mask Help:
      | Sends signal(s) from Simulink to the Sensor World.
      | 
      | - Port Name [-]: specifies the name of the output terminal of the Simulink block.
      | - Index [-]: specifies the start position in the output vector sent to the Sensor World
      | - Port dimensions [-]: specifies the width (number of scalars) of the output port
      | - Upload period [s]: specifies the upload period (in seconds) of the port.
      mask Display: port_label('input', 1, PortName)
  wires:
  Demux/5 -> velRPY/1(Y)
  Demux/4 -> RPY/1(Y)
  Demux/3 -> Acceleration/1(Y)
  Demux/2 -> Velocity/1(Y)
  Demux/1 -> Position/1(Y)
  State/1 -> state2FullState/1
  state2FullState/1 -> Demux/1
  iniVEHposition wrtGLOB [m]/1 -> state2FullState/2
  iniBODYAngles wrtVEH [rad]/1 -> state2FullState/3
  iniVEHAngles wrtGLOB [rad]/1 -> state2FullState/4

== system Demo_LaneKeeping_cs/SetActuators ==
  Bus Creator : BusCreator  Inputs=1
  Data Store Read : DataStoreRead  DataStoreName=SimCoreActuators  SampleTime=TimeStep
  SendActuators : M-S-Function  FunctionName=SendActuatorsBlock  Parameters=TimeStep NrOfActuators
  dummy : Outport
  tag scope: SimCoreInfo=global
  wires:
  Bus Creator/1 -> [SimCoreInfo]  "SimCore"
  SendActuators/2 -> Bus Creator/1  "ComputationTime[s]"
  SendActuators/1 -> dummy/1
  Data Store Read/1 -> SendActuators/1

== system Demo_LaneKeeping_cs/SimCoreInfo ==
  Bus Selector : BusSelector  OutputSignals=ComputationTime[s]
  Time : Scope
  wires:
  Bus Selector/1 -> Time/1  "<ComputationTime[s]>"
  [SimCoreInfo] -> Bus Selector/1

== system Demo_LaneKeeping_cs/VISUSteer_Mazda_RX8_1 ==
  Steer : Inport
  Demux3 : Demux  Outputs=[1 1]
  Saturation : Saturate  UpperLimit=30  LowerLimit=-5
  Saturation1 : Saturate  UpperLimit=720  LowerLimit=-720
  conv_SteeringColumn : Subsystem
  conv_SteeringWheel : Subsystem
  visu_SteeringColumn : Subsystem  mask(ToSensorWorld){PortName=visu_SteeringColumn_0, PortIndex=47, PortWidth=4, TimeStep=1/20}
      mask prompts: PortName "Port Name [-]"; PortIndex "Index [-]"; PortWidth "Port Dimensions [-]"; TimeStep "Upload Period [s]"
      mask help: Sends signal(s) from Simulink to the Sensor World
      mask Help:
      | Sends signal(s) from Simulink to the Sensor World.
      | 
      | - Port Name [-]: specifies the name of the output terminal of the Simulink block.
      | - Index [-]: specifies the start position in the output vector sent to the Sensor World
      | - Port dimensions [-]: specifies the width (number of scalars) of the output port
      | - Upload period [s]: specifies the upload period (in seconds) of the port.
      mask Display: port_label('input', 1, PortName)
  visu_SteeringWheel : Subsystem  mask(ToSensorWorld){PortName=visu_SteeringWheel_0, PortIndex=43, PortWidth=4, TimeStep=1/20}
      mask prompts: PortName "Port Name [-]"; PortIndex "Index [-]"; PortWidth "Port Dimensions [-]"; TimeStep "Upload Period [s]"
      mask help: Sends signal(s) from Simulink to the Sensor World
      mask Help:
      | Sends signal(s) from Simulink to the Sensor World.
      | 
      | - Port Name [-]: specifies the name of the output terminal of the Simulink block.
      | - Index [-]: specifies the start position in the output vector sent to the Sensor World
      | - Port dimensions [-]: specifies the width (number of scalars) of the output port
      | - Upload period [s]: specifies the upload period (in seconds) of the port.
      mask Display: port_label('input', 1, PortName)
  wires:
  conv_SteeringColumn/1(QuaternionVisu [rad]) -> visu_SteeringColumn/1(Y)
  conv_SteeringWheel/1(QuaternionVisu [rad]) -> visu_SteeringWheel/1(Y)
  Demux3/2 -> Saturation/1
  Demux3/1 -> Saturation1/1
  Saturation1/1 -> conv_SteeringWheel/1(angle [deg])
  Saturation/1 -> conv_SteeringColumn/1(angle [deg])
  Steer/1 -> Demux3/1

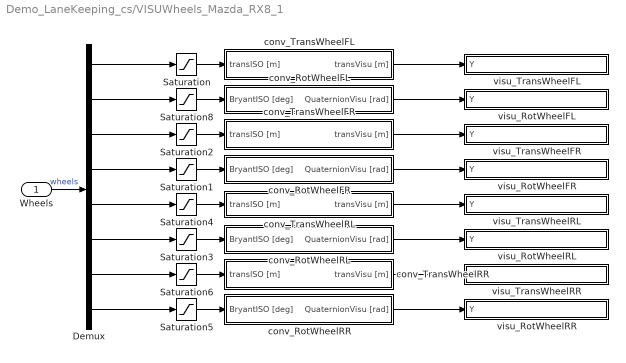
== system Demo_LaneKeeping_cs/VISUWheels_Mazda_RX8_1 ==
  Wheels : Inport
  Demux : Demux  Outputs=[3 3 3 3 3 3 3 3]
  Saturation{,2,4,6} (4 alike) : Saturate  UpperLimit=[0.2 0.2 0.5]  LowerLimit=[-0.2 -0.2 -0.5]
  Saturation{1,3,5,8} (4 alike) : Saturate  UpperLimit=[30 inf 30]  LowerLimit=[-30 -inf -30]
  conv_RotWheelFL : Subsystem
  conv_RotWheelFR : Subsystem
  conv_RotWheelRL : Subsystem
  conv_RotWheelRR : Subsystem
  conv_TransWheelFL : Subsystem  mask(Translation node configuration){tp=Front-Left Wheel, gains=off, Gain_xISO=1, Gain_yISO=1, Gain_zISO=1}
      mask prompts: tp "Type"; gains "Edit scaling factors?"; Gain_xISO "Scaling factor in x-direction (ISO-convention)"; Gain_yISO "Scaling factor in y-direction (ISO-convention)"; Gain_zISO "Scaling factor in z-direction (ISO-convention)"
      mask init:
      | Visu_ini_param('Mazda_RX8',tp);
      mask TypeOptions tp: Front-Left Wheel | Front-Right Wheel | Rear-Left Wheel | Rear-Right Wheel | Left Seat | Right Seat
      mask Callback gains:
      | if strcmp(get_param(gcb, 'gains'),'on')
      |     set_param(gcb,'MaskVisibilities',{'on','on','on','on','on'})
      | else
      |     set_param(gcb,'MaskVisibilities',{'on','on','off','off','off'})
      | end
  conv_TransWheelFR : Subsystem  mask(Translation node configuration){tp=Front-Right Wheel, gains=off, Gain_xISO=1, Gain_yISO=1, Gain_zISO=1}
      mask prompts: tp "Type"; gains "Edit scaling factors?"; Gain_xISO "Scaling factor in x-direction (ISO-convention)"; Gain_yISO "Scaling factor in y-direction (ISO-convention)"; Gain_zISO "Scaling factor in z-direction (ISO-convention)"
      mask init:
      | Visu_ini_param('Mazda_RX8',tp);
      mask TypeOptions tp: Front-Left Wheel | Front-Right Wheel | Rear-Left Wheel | Rear-Right Wheel | Left Seat | Right Seat
      mask Callback gains:
      | if strcmp(get_param(gcb, 'gains'),'on')
      |     set_param(gcb,'MaskVisibilities',{'on','on','on','on','on'})
      | else
      |     set_param(gcb,'MaskVisibilities',{'on','on','off','off','off'})
      | end
  conv_TransWheelRL : Subsystem  mask(Translation node configuration){tp=Rear-Left Wheel, gains=off, Gain_xISO=1, Gain_yISO=1, Gain_zISO=1}
      mask prompts: tp "Type"; gains "Edit scaling factors?"; Gain_xISO "Scaling factor in x-direction (ISO-convention)"; Gain_yISO "Scaling factor in y-direction (ISO-convention)"; Gain_zISO "Scaling factor in z-direction (ISO-convention)"
      mask init:
      | Visu_ini_param('Mazda_RX8',tp);
      mask TypeOptions tp: Front-Left Wheel | Front-Right Wheel | Rear-Left Wheel | Rear-Right Wheel | Left Seat | Right Seat
      mask Callback gains:
      | if strcmp(get_param(gcb, 'gains'),'on')
      |     set_param(gcb,'MaskVisibilities',{'on','on','on','on','on'})
      | else
      |     set_param(gcb,'MaskVisibilities',{'on','on','off','off','off'})
      | end
  conv_TransWheelRR : Subsystem  mask(Translation node configuration){tp=Rear-Right Wheel, gains=off, Gain_xISO=1, Gain_yISO=1, Gain_zISO=1}
      mask prompts: tp "Type"; gains "Edit scaling factors?"; Gain_xISO "Scaling factor in x-direction (ISO-convention)"; Gain_yISO "Scaling factor in y-direction (ISO-convention)"; Gain_zISO "Scaling factor in z-direction (ISO-convention)"
      mask init:
      | Visu_ini_param('Mazda_RX8',tp);
      mask TypeOptions tp: Front-Left Wheel | Front-Right Wheel | Rear-Left Wheel | Rear-Right Wheel | Left Seat | Right Seat
      mask Callback gains:
      | if strcmp(get_param(gcb, 'gains'),'on')
      |     set_param(gcb,'MaskVisibilities',{'on','on','on','on','on'})
      | else
      |     set_param(gcb,'MaskVisibilities',{'on','on','off','off','off'})
      | end
  visu_RotWheelFL : Subsystem  mask(ToSensorWorld){PortName=visu_RotWheelFL_0, PortIndex=18, PortWidth=4, TimeStep=1/20}
      mask prompts: PortName "Port Name [-]"; PortIndex "Index [-]"; PortWidth "Port Dimensions [-]"; TimeStep "Upload Period [s]"
      mask help: Sends signal(s) from Simulink to the Sensor World
      mask Help:
      | Sends signal(s) from Simulink to the Sensor World.
      | 
      | - Port Name [-]: specifies the name of the output terminal of the Simulink block.
      | - Index [-]: specifies the start position in the output vector sent to the Sensor World
      | - Port dimensions [-]: specifies the width (number of scalars) of the output port
      | - Upload period [s]: specifies the upload period (in seconds) of the port.
      mask Display: port_label('input', 1, PortName)
  visu_RotWheelFR : Subsystem  mask(ToSensorWorld){PortName=visu_RotWheelFR_0, PortIndex=25, PortWidth=4, TimeStep=1/20}
      mask prompts: PortName "Port Name [-]"; PortIndex "Index [-]"; PortWidth "Port Dimensions [-]"; TimeStep "Upload Period [s]"
      mask help: Sends signal(s) from Simulink to the Sensor World
      mask Help:
      | Sends signal(s) from Simulink to the Sensor World.
      | 
      | - Port Name [-]: specifies the name of the output terminal of the Simulink block.
      | - Index [-]: specifies the start position in the output vector sent to the Sensor World
      | - Port dimensions [-]: specifies the width (number of scalars) of the output port
      | - Upload period [s]: specifies the upload period (in seconds) of the port.
      mask Display: port_label('input', 1, PortName)
  visu_RotWheelRL : Subsystem  mask(ToSensorWorld){PortName=visu_RotWheelRL_0, PortIndex=32, PortWidth=4, TimeStep=1/20}
      mask prompts: PortName "Port Name [-]"; PortIndex "Index [-]"; PortWidth "Port Dimensions [-]"; TimeStep "Upload Period [s]"
      mask help: Sends signal(s) from Simulink to the Sensor World
      mask Help:
      | Sends signal(s) from Simulink to the Sensor World.
      | 
      | - Port Name [-]: specifies the name of the output terminal of the Simulink block.
      | - Index [-]: specifies the start position in the output vector sent to the Sensor World
      | - Port dimensions [-]: specifies the width (number of scalars) of the output port
      | - Upload period [s]: specifies the upload period (in seconds) of the port.
      mask Display: port_label('input', 1, PortName)
  visu_RotWheelRR : Subsystem  mask(ToSensorWorld){PortName=visu_RotWheelRR_0, PortIndex=39, PortWidth=4, TimeStep=1/20}
      mask prompts: PortName "Port Name [-]"; PortIndex "Index [-]"; PortWidth "Port Dimensions [-]"; TimeStep "Upload Period [s]"
      mask help: Sends signal(s) from Simulink to the Sensor World
      mask Help:
      | Sends signal(s) from Simulink to the Sensor World.
      | 
      | - Port Name [-]: specifies the name of the output terminal of the Simulink block.
      | - Index [-]: specifies the start position in the output vector sent to the Sensor World
      | - Port dimensions [-]: specifies the width (number of scalars) of the output port
      | - Upload period [s]: specifies the upload period (in seconds) of the port.
      mask Display: port_label('input', 1, PortName)
  visu_TransWheelFL : Subsystem  mask(ToSensorWorld){PortName=visu_TransWheelFL_0, PortIndex=15, PortWidth=3, TimeStep=1/20}
      mask prompts: PortName "Port Name [-]"; PortIndex "Index [-]"; PortWidth "Port Dimensions [-]"; TimeStep "Upload Period [s]"
      mask help: Sends signal(s) from Simulink to the Sensor World
      mask Help:
      | Sends signal(s) from Simulink to the Sensor World.
      | 
      | - Port Name [-]: specifies the name of the output terminal of the Simulink block.
      | - Index [-]: specifies the start position in the output vector sent to the Sensor World
      | - Port dimensions [-]: specifies the width (number of scalars) of the output port
      | - Upload period [s]: specifies the upload period (in seconds) of the port.
      mask Display: port_label('input', 1, PortName)
  visu_TransWheelFR : Subsystem  mask(ToSensorWorld){PortName=visu_TransWheelFR_0, PortIndex=22, PortWidth=3, TimeStep=1/20}
      mask prompts: PortName "Port Name [-]"; PortIndex "Index [-]"; PortWidth "Port Dimensions [-]"; TimeStep "Upload Period [s]"
      mask help: Sends signal(s) from Simulink to the Sensor World
      mask Help:
      | Sends signal(s) from Simulink to the Sensor World.
      | 
      | - Port Name [-]: specifies the name of the output terminal of the Simulink block.
      | - Index [-]: specifies the start position in the output vector sent to the Sensor World
      | - Port dimensions [-]: specifies the width (number of scalars) of the output port
      | - Upload period [s]: specifies the upload period (in seconds) of the port.
      mask Display: port_label('input', 1, PortName)
  visu_TransWheelRL : Subsystem  mask(ToSensorWorld){PortName=visu_TransWheelRL_0, PortIndex=29, PortWidth=3, TimeStep=1/20}
      mask prompts: PortName "Port Name [-]"; PortIndex "Index [-]"; PortWidth "Port Dimensions [-]"; TimeStep "Upload Period [s]"
      mask help: Sends signal(s) from Simulink to the Sensor World
      mask Help:
      | Sends signal(s) from Simulink to the Sensor World.
      | 
      | - Port Name [-]: specifies the name of the output terminal of the Simulink block.
      | - Index [-]: specifies the start position in the output vector sent to the Sensor World
      | - Port dimensions [-]: specifies the width (number of scalars) of the output port
      | - Upload period [s]: specifies the upload period (in seconds) of the port.
      mask Display: port_label('input', 1, PortName)
  visu_TransWheelRR : Subsystem  mask(ToSensorWorld){PortName=visu_TransWheelRR_0, PortIndex=36, PortWidth=3, TimeStep=1/20}
      mask prompts: PortName "Port Name [-]"; PortIndex "Index [-]"; PortWidth "Port Dimensions [-]"; TimeStep "Upload Period [s]"
      mask help: Sends signal(s) from Simulink to the Sensor World
      mask Help:
      | Sends signal(s) from Simulink to the Sensor World.
      | 
      | - Port Name [-]: specifies the name of the output terminal of the Simulink block.
      | - Index [-]: specifies the start position in the output vector sent to the Sensor World
      | - Port dimensions [-]: specifies the width (number of scalars) of the output port
      | - Upload period [s]: specifies the upload period (in seconds) of the port.
      mask Display: port_label('input', 1, PortName)
  wires:
  conv_RotWheelRR/1(QuaternionVisu [rad]) -> visu_RotWheelRR/1(Y)
  conv_TransWheelRR/1(transVisu [m]) -> visu_TransWheelRR/1(Y)
  conv_RotWheelRL/1(QuaternionVisu [rad]) -> visu_RotWheelRL/1(Y)
  conv_TransWheelRL/1(transVisu [m]) -> visu_TransWheelRL/1(Y)
  conv_RotWheelFR/1(QuaternionVisu [rad]) -> visu_RotWheelFR/1(Y)
  conv_TransWheelFR/1(transVisu [m]) -> visu_TransWheelFR/1(Y)
  conv_RotWheelFL/1(QuaternionVisu [rad]) -> visu_RotWheelFL/1(Y)
  conv_TransWheelFL/1(transVisu [m]) -> visu_TransWheelFL/1(Y)
  Demux/8 -> Saturation5/1
  Demux/7 -> Saturation6/1
  Demux/6 -> Saturation3/1
  Demux/5 -> Saturation4/1
  Demux/4 -> Saturation1/1
  Demux/3 -> Saturation2/1
  Demux/2 -> Saturation8/1
  Demux/1 -> Saturation/1
  Saturation5/1 -> conv_RotWheelRR/1(BryantISO [deg])
  Saturation6/1 -> conv_TransWheelRR/1(transISO [m])
  Saturation3/1 -> conv_RotWheelRL/1(BryantISO [deg])
  Saturation4/1 -> conv_TransWheelRL/1(transISO [m])
  Saturation1/1 -> conv_RotWheelFR/1(BryantISO [deg])
  Saturation2/1 -> conv_TransWheelFR/1(transISO [m])
  Saturation8/1 -> conv_RotWheelFL/1(BryantISO [deg])
  Saturation/1 -> conv_TransWheelFL/1(transISO [m])
  Wheels/1 -> Demux/1  "wheels"

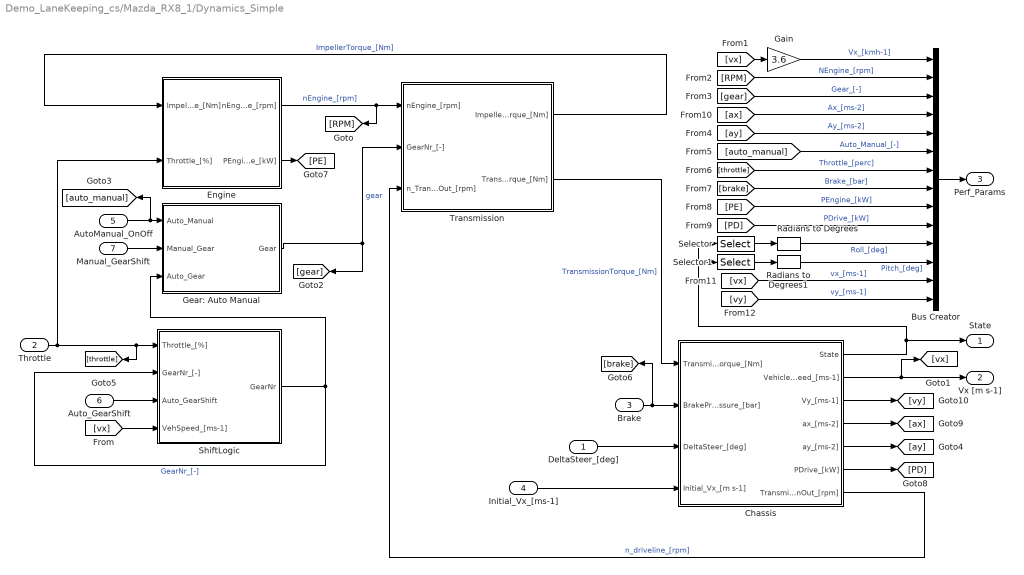
== system Demo_LaneKeeping_cs/Mazda_RX8_1/Dynamics_Simple ==
  DeltaSteer_[deg] : Inport
  Throttle : Inport  Port=2
  Brake : Inport  Port=3
  Initial_Vx_[ms-1] : Inport  Port=4
  AutoManual_OnOff : Inport  Port=5
  Auto_GearShift : Inport  Port=6
  Manual_GearShift : Inport  Port=7
  Bus Creator : BusCreator  Inputs=14
  Chassis : Subsystem
      mask Display: image(imread('Chassis.png'));
  Engine : Subsystem
      mask Display: image(imread('Engine.png'));
  Gain : Gain  Gain=3.6
  Gear: Auto Manual : Subsystem
  Radians to Degrees : simulink_extras/Transformations/Radians to Degrees
  Radians to Degrees1 : simulink_extras/Transformations/Radians to Degrees
  Selector : Selector  InputPortWidth=9  IndexOptions=Index vector (dialog)  Indices=7  OutputSizes=1
  Selector1 : Selector  InputPortWidth=9  IndexOptions=Index vector (dialog)  Indices=8  OutputSizes=1
  ShiftLogic : Subsystem
      mask Display: image(imread('Gearshift.png'));
  Transmission : Subsystem
      mask Display: image(imread('Transmission.png'));
  State : Outport
  Vx [m s-1] : Outport  Port=2
  Perf_Params : Outport  Port=3
  wires:
  [vy] -> Bus Creator/14  "vy_[ms-1]"
  [vx] -> Bus Creator/13  "vx_[ms-1]"
  Chassis/7(TransmissionOut_[rpm]) -> Transmission/3(n_TransmissionOut_[rpm])  "n_driveline_[rpm]"
  Chassis/6(PDrive_[kW]) -> [PD]
  Chassis/5(ay_[ms-2]) -> [ay]
  Chassis/4(ax_[ms-2]) -> [ax]
  Chassis/3(Vy_[ms-1]) -> [vy]
  [vx] -> ShiftLogic/4(VehSpeed_[ms-1])
  Gear: Auto Manual/1(Gear) -> Transmission/2(GearNr_[-]), [gear]  "gear"
  Manual_GearShift/1 -> Gear: Auto Manual/2(Manual_Gear)
  AutoManual_OnOff/1 -> Gear: Auto Manual/1(Auto_Manual), [auto_manual]
  Chassis/2(VehicleSpeed_[ms-1]) -> [vx], Vx [m s-1]/1
  Auto_GearShift/1 -> ShiftLogic/3(Auto_GearShift)
  Throttle/1 -> Engine/2(Throttle_[%]), ShiftLogic/1(Throttle_[%]), [throttle]
  Initial_Vx_[ms-1]/1 -> Chassis/4(Initial_Vx_[m s-1])
  DeltaSteer_[deg]/1 -> Chassis/3(DeltaSteer_[deg])
  Chassis/1(State) -> State/1, Selector/1, Selector1/1
  Brake/1 -> [brake], Chassis/2(BrakePressure_[bar])
  Engine/1(nEngine_[rpm]) -> [RPM], Transmission/1(nEngine_[rpm])  "nEngine_[rpm]"
  ShiftLogic/1(GearNr) -> Gear: Auto Manual/3(Auto_Gear), ShiftLogic/2(GearNr_[-])  "GearNr_[-]"
  Transmission/2(TransmissionTorque_[Nm]) -> Chassis/1(TransmissionTorque_[Nm])  "TransmissionTorque_[Nm]"
  Transmission/1(ImpellerTorque_[Nm]) -> Engine/1(ImpellerTorque_[Nm])  "ImpellerTorque_[Nm]"
  Gain/1 -> Bus Creator/1  "Vx_[kmh-1]"
  [RPM] -> Bus Creator/2  "NEngine_[rpm]"
  [gear] -> Bus Creator/3  "Gear_[-]"
  [ay] -> Bus Creator/5  "Ay_[ms-2]"
  [auto_manual] -> Bus Creator/6  "Auto_Manual_[-]"
  [throttle] -> Bus Creator/7  "Throttle_[perc]"
  [brake] -> Bus Creator/8  "Brake_[bar]"
  Engine/2(PEngine_[kW]) -> [PE]
  Bus Creator/1 -> Perf_Params/1
  [PE] -> Bus Creator/9  "PEngine_[kW]"
  Radians to Degrees/1 -> Bus Creator/11  "Roll_[deg]"
  Radians to Degrees1/1 -> Bus Creator/12  "Pitch_[deg]"
  [PD] -> Bus Creator/10  "PDrive_[kW]"
  Selector/1 -> Radians to Degrees/1
  Selector1/1 -> Radians to Degrees1/1
  [vx] -> Gain/1
  [ax] -> Bus Creator/4  "Ax_[ms-2]"

== system Demo_LaneKeeping_cs/Mazda_RX8_1/Lane Keeping Algorithm ==
  Sensor Data : Inport
  Add : Sum
  Add1 : Sum
  Add2 : Sum
  Bus Selector : BusSelector  OutputSignals=ScanAtSensor.SliceCenterCoordsX,ScanAtSensor.SliceCenterCoordsY,ScanAtDistance1.SliceCenterCoordsX,ScanAtDistance1.SliceCenterCoordsY,ScanAtSensor.RightLaneIntersection1.WorldCoordinateX,ScanAtSensor.RightLaneIntersection1.WorldCoordinateY,ScanAtDistance1.RightLaneIntersection1.WorldCoordinateX,ScanAtDistance1.RightLaneIntersection1.WorldCoordinateY
  Bus Selector1 : BusSelector  OutputSignals=ScanAtDistance1.LeftLaneIntersection1.DistanceFromScanCenter,ScanAtDistance1.RightLaneIntersection1.DistanceFromScanCenter
  Constant : Constant  Value=-0.5
  Divide : Product  Inputs=/*
  Scaler1 : Constant  Value=1250
  Scaler2 : Gain  Gain=-250
  "angular error " : M-S-Function  FunctionName=angular_error_msfun
      mask Display:
      | port_label('input',1,'cx1')
      | port_label('input',2,'cy1')
      | port_label('input',3,'cx2')
      | port_label('input',4,'cy2')
      | port_label('input',5,'lsx1')
      | port_label('input',6,'lsy1')
      | port_label('input',7,'lsx2')
      | port_label('input',8,'lsy2')
      | port_label('input',9,'scaler')
      | port_label('output',1,'angle')
  Steering Angle : Outport
  wires:
  Sensor Data/1 -> Bus Selector1/1, Bus Selector/1
  Bus Selector1/1 -> Add/1  "<DistanceFromScanCenter>"
  Bus Selector1/2 -> Divide/2, Add/2  "<DistanceFromScanCenter>"
  Add/1 -> Divide/1
  Divide/1 -> Add1/2
  Constant/1 -> Add1/1
  Add1/1 -> Scaler2/1
  Scaler2/1 -> Add2/2
  Add2/1 -> Steering Angle/1
  Bus Selector/1 -> "angular error "/1  "<SliceCenterCoordsX>"
  Bus Selector/2 -> "angular error "/2  "<SliceCenterCoordsY>"
  Bus Selector/3 -> "angular error "/3  "<SliceCenterCoordsX>"
  Bus Selector/4 -> "angular error "/4  "<SliceCenterCoordsY>"
  Bus Selector/5 -> "angular error "/5  "<WorldCoordinateX>"
  Bus Selector/6 -> "angular error "/6  "<WorldCoordinateY>"
  Bus Selector/7 -> "angular error "/7  "<WorldCoordinateX>"
  Bus Selector/8 -> "angular error "/8  "<WorldCoordinateY>"
  "angular error "/1 -> Add2/1
  Scaler1/1 -> "angular error "/9

== system Demo_LaneKeeping_cs/Mazda_RX8_1/SELF_Demux ==
  SELF : Inport
  Demux1 : Demux  Outputs=3
  Demux2 : Demux  Outputs=3
  Demux3 : Demux  Outputs=[3 3 1 1]
  Demux4 : Demux  Outputs=3
  Gain : Gain  Gain=180/pi
  Gain1 : Gain  Gain=180/pi
  Selector : Selector  InputPortWidth=3  IndexOptions=Index vector (dialog)  Indices=[3]  OutputSizes=1
  compas converter : Subsystem
  xyz2GPS : PreScanUsefulBlocks/xyz2GPS  CoordinateCount=1  GPS_base=[0.000000 0.000000 0.000]
  x [m] : Outport
  y [m] : Outport  Port=2
  z [m] : Outport  Port=3
  rotx [deg] : Outport  Port=4
  roty [deg] : Outport  Port=5
  rotz [deg] : Outport  Port=6
  GPS lat [deg] : Outport  Port=7
  GPS long [deg] : Outport  Port=8
  GPS alt [m] : Outport  Port=9
  velocity [m/s] : Outport  Port=10
  heading [deg] : Outport  Port=11
  yaw rate [deg/s] : Outport  Port=12
  wires:
  Demux3/4 -> Gain1/1
  Gain1/1 -> yaw rate [deg/s]/1
  Demux3/3 -> velocity [m/s]/1
  compas converter/1(heading [deg]) -> heading [deg]/1
  xyz2GPS/1 -> Demux4/1
  Demux4/3 -> GPS alt [m]/1
  Demux4/2 -> GPS long [deg]/1
  Demux4/1 -> GPS lat [deg]/1
  Demux3/2 -> Gain/1, Selector/1
  Demux3/1 -> xyz2GPS/1, Demux1/1
  SELF/1 -> Demux3/1
  Demux2/3 -> rotz [deg]/1
  Demux2/2 -> roty [deg]/1
  Demux2/1 -> rotx [deg]/1
  Demux1/3 -> z [m]/1
  Demux1/2 -> y [m]/1
  Demux1/1 -> x [m]/1
  Gain/1 -> Demux2/1
  Selector/1 -> compas converter/1(rotz [rad])

== system Demo_LaneKeeping_cs/Mazda_RX8_1/VISUSteer_Mux ==
  Column [deg] : Inport
  Steer [deg] : Inport  Port=2
  Mux2 : Mux  Inputs=2
  Steer : Outport
  wires:
  Column [deg]/1 -> Mux2/2
  Mux2/1 -> Steer/1
  Steer [deg]/1 -> Mux2/1

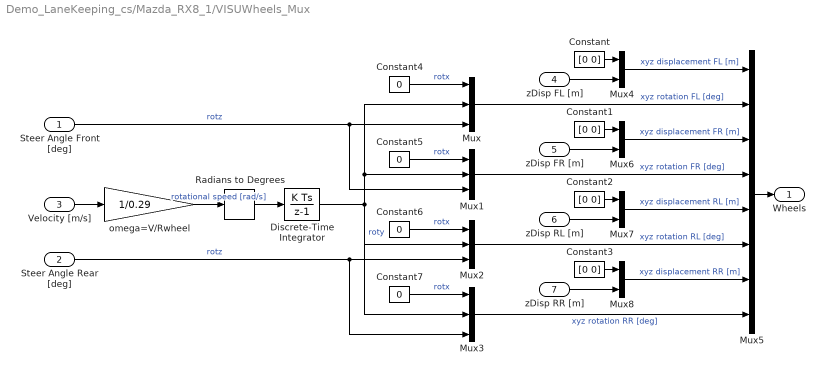
== system Demo_LaneKeeping_cs/Mazda_RX8_1/VISUWheels_Mux ==
  Steer Angle Front [deg] : Inport  SampleTime=TimeStep
  Steer Angle Rear [deg] : Inport  Port=2  SampleTime=TimeStep
  Velocity [m/s] : Inport  Port=3  SampleTime=TimeStep
  zDisp FL [m] : Inport  Port=4  SampleTime=TimeStep
  zDisp FR [m] : Inport  Port=5  SampleTime=TimeStep
  zDisp RL [m] : Inport  Port=6  SampleTime=TimeStep
  zDisp RR [m] : Inport  Port=7  SampleTime=TimeStep
  Constant{,1..3} (4 alike) : Constant  Value=[0 0]  SampleTime=TimeStep
  Constant{4..7} (4 alike) : Constant  Value=0  SampleTime=TimeStep
  Discrete-Time Integrator : DiscreteIntegrator  SampleTime=TimeStep  ICPrevOutput=DiscIntNeverNeededParam  ICPrevScaledInput=DiscIntNeverNeededParam
  Mux{,1..3} (4 alike) : Mux  Inputs=3
  Mux{4,6..8} (4 alike) : Mux  Inputs=[2 1]
  Mux5 : Mux  Inputs=[3 3 3 3 3 3 3 3]
  Radians to Degrees : simulink_extras/Transformations/Radians to Degrees
  omega=V/Rwheel : Gain  Gain=1/0.29
  Wheels : Outport
  wires:
  Mux7/1 -> Mux5/5  "xyz displacement RL [m]"
  Discrete-Time Integrator/1 -> Mux/2, Mux1/2, Mux2/2, Mux3/2  "roty"
  Radians to Degrees/1 -> Discrete-Time Integrator/1
  Constant7/1 -> Mux3/1  "rotx"
  Constant6/1 -> Mux2/1  "rotx"
  Constant5/1 -> Mux1/1  "rotx"
  Constant4/1 -> Mux/1  "rotx"
  Steer Angle Front [deg]/1 -> Mux1/3, Mux/3  "rotz"
  Steer Angle Rear [deg]/1 -> Mux3/3, Mux2/3  "rotz"
  Mux8/1 -> Mux5/7  "xyz displacement RR [m]"
  Mux6/1 -> Mux5/3  "xyz displacement FR [m]"
  Mux4/1 -> Mux5/1  "xyz displacement FL [m]"
  Constant3/1 -> Mux8/1
  Constant2/1 -> Mux7/1
  Constant1/1 -> Mux6/1
  Constant/1 -> Mux4/1
  zDisp RR [m]/1 -> Mux8/2
  zDisp RL [m]/1 -> Mux7/2
  zDisp FR [m]/1 -> Mux6/2
  zDisp FL [m]/1 -> Mux4/2
  Mux5/1 -> Wheels/1
  omega=V/Rwheel/1 -> Radians to Degrees/1  "rotational speed [rad/s]"
  Velocity [m/s]/1 -> omega=V/Rwheel/1
  Mux1/1 -> Mux5/4  "xyz rotation FR [deg]"
  Mux/1 -> Mux5/2  "xyz rotation FL [deg]"
  Mux3/1 -> Mux5/8  "xyz rotation RR [deg]"
  Mux2/1 -> Mux5/6  "xyz rotation RL [deg]"

== system Demo_LaneKeeping_cs/STATE_Mazda_RX8_1/Acceleration ==
  Y : Inport
  Assignment : Assignment  IndexMode=Zero-based  SampleTime=TimeStep  IndexOptions=Starting index (dialog)  Indices=PortIndex  OutputSizes=[1 1]
  Data Store Read : DataStoreRead  DataStoreName=SimCoreActuators  SampleTime=TimeStep
  Data Store Write : DataStoreWrite  DataStoreName=SimCoreActuators
  wires:
  Assignment/1 -> Data Store Write/1
  Data Store Read/1 -> Assignment/1
  Y/1 -> Assignment/2

== system Demo_LaneKeeping_cs/STATE_Mazda_RX8_1/Position ==
  Y : Inport
  Assignment : Assignment  IndexMode=Zero-based  SampleTime=TimeStep  IndexOptions=Starting index (dialog)  Indices=PortIndex  OutputSizes=[1 1]
  Data Store Read : DataStoreRead  DataStoreName=SimCoreActuators  SampleTime=TimeStep
  Data Store Write : DataStoreWrite  DataStoreName=SimCoreActuators
  wires:
  Y/1 -> Assignment/2
  Data Store Read/1 -> Assignment/1
  Assignment/1 -> Data Store Write/1

== system Demo_LaneKeeping_cs/STATE_Mazda_RX8_1/RPY ==
  Y : Inport
  Assignment : Assignment  IndexMode=Zero-based  SampleTime=TimeStep  IndexOptions=Starting index (dialog)  Indices=PortIndex  OutputSizes=[1 1]
  Data Store Read : DataStoreRead  DataStoreName=SimCoreActuators  SampleTime=TimeStep
  Data Store Write : DataStoreWrite  DataStoreName=SimCoreActuators
  wires:
  Assignment/1 -> Data Store Write/1
  Data Store Read/1 -> Assignment/1
  Y/1 -> Assignment/2

== system Demo_LaneKeeping_cs/STATE_Mazda_RX8_1/Velocity ==
  Y : Inport
  Assignment : Assignment  IndexMode=Zero-based  SampleTime=TimeStep  IndexOptions=Starting index (dialog)  Indices=PortIndex  OutputSizes=[1 1]
  Data Store Read : DataStoreRead  DataStoreName=SimCoreActuators  SampleTime=TimeStep
  Data Store Write : DataStoreWrite  DataStoreName=SimCoreActuators
  wires:
  Assignment/1 -> Data Store Write/1
  Data Store Read/1 -> Assignment/1
  Y/1 -> Assignment/2

== system Demo_LaneKeeping_cs/STATE_Mazda_RX8_1/velRPY ==
  Y : Inport
  Assignment : Assignment  IndexMode=Zero-based  SampleTime=TimeStep  IndexOptions=Starting index (dialog)  Indices=PortIndex  OutputSizes=[1 1]
  Data Store Read : DataStoreRead  DataStoreName=SimCoreActuators  SampleTime=TimeStep
  Data Store Write : DataStoreWrite  DataStoreName=SimCoreActuators
  wires:
  Assignment/1 -> Data Store Write/1
  Data Store Read/1 -> Assignment/1
  Y/1 -> Assignment/2

== system Demo_LaneKeeping_cs/VISUSteer_Mazda_RX8_1/conv_SteeringColumn ==
  angle [deg] : Inport
  Constant13 : Constant  Value=[0 1 0]
  Mux8 : Mux  Inputs=2
  deg2rad : Gain  Gain=pi/180
  QuaternionVisu [rad] : Outport
  wires:
  deg2rad/1 -> Mux8/2
  Constant13/1 -> Mux8/1
  Mux8/1 -> QuaternionVisu [rad]/1
  angle [deg]/1 -> deg2rad/1

== system Demo_LaneKeeping_cs/VISUSteer_Mazda_RX8_1/conv_SteeringWheel ==
  angle [deg] : Inport
  Constant13 : Constant  Value=[-1 0 0]
  Mux8 : Mux  Inputs=2
  deg2rad : Gain  Gain=pi/180
  QuaternionVisu [rad] : Outport
  wires:
  deg2rad/1 -> Mux8/2
  Constant13/1 -> Mux8/1
  Mux8/1 -> QuaternionVisu [rad]/1
  angle [deg]/1 -> deg2rad/1

== system Demo_LaneKeeping_cs/VISUSteer_Mazda_RX8_1/visu_SteeringColumn ==
  Y : Inport
  Assignment : Assignment  IndexMode=Zero-based  SampleTime=TimeStep  IndexOptions=Starting index (dialog)  Indices=PortIndex  OutputSizes=[1 1]
  Data Store Read : DataStoreRead  DataStoreName=SimCoreActuators  SampleTime=TimeStep
  Data Store Write : DataStoreWrite  DataStoreName=SimCoreActuators
  wires:
  Assignment/1 -> Data Store Write/1
  Data Store Read/1 -> Assignment/1
  Y/1 -> Assignment/2

== system Demo_LaneKeeping_cs/VISUSteer_Mazda_RX8_1/visu_SteeringWheel ==
  Y : Inport
  Assignment : Assignment  IndexMode=Zero-based  SampleTime=TimeStep  IndexOptions=Starting index (dialog)  Indices=PortIndex  OutputSizes=[1 1]
  Data Store Read : DataStoreRead  DataStoreName=SimCoreActuators  SampleTime=TimeStep
  Data Store Write : DataStoreWrite  DataStoreName=SimCoreActuators
  wires:
  Assignment/1 -> Data Store Write/1
  Data Store Read/1 -> Assignment/1
  Y/1 -> Assignment/2

== system Demo_LaneKeeping_cs/VISUWheels_Mazda_RX8_1/conv_RotWheelFL ==
  BryantISO [deg] : Inport
  Fcn10 : Fcn  Expr=cos(u(1))*sin(u(3))+sin(u(1))*sin(u(2))*cos(u(3))
  Fcn11 : Fcn  Expr=sin(u(1))*sin(u(3))-cos(u(1))*sin(u(2))*cos(u(3))
  Fcn12 : Fcn  Expr=-cos(u(2))*sin(u(3))
  Fcn13 : Fcn  Expr=cos(u(1))*cos(u(3))-sin(u(1))*sin(u(2))*sin(u(3))
  Fcn14 : Fcn  Expr=sin(u(1))*cos(u(3))+cos(u(1))*sin(u(2))*sin(u(3))
  Fcn15 : Fcn  Expr=sin(u(2))
  Fcn16 : Fcn  Expr=-sin(u(1))*cos(u(2))
  Fcn17 : Fcn  Expr=cos(u(1))*cos(u(2))
  Fcn9 : Fcn  Expr=cos(u(2))*cos(u(3))
  Mux1 : Mux  Inputs=9
  RotMat2AxisAngle : Subsystem
  deg2rad : Gain  Gain=pi/180
  xyz 2 zxy : Selector  InputPortWidth=3  IndexOptions=Index vector (dialog)  Indices=[3 1 2]  OutputSizes=1
  zxy 2 xyz : Selector  InputPortWidth=4  IndexOptions=Index vector (dialog)  Indices=[2 3 1 4]  OutputSizes=1
  QuaternionVisu [rad] : Outport
  wires:
  zxy 2 xyz/1 -> QuaternionVisu [rad]/1
  xyz 2 zxy/1 -> deg2rad/1
  deg2rad/1 -> Fcn17/1, Fcn16/1, Fcn15/1, Fcn14/1, Fcn13/1, Fcn12/1, Fcn11/1, Fcn10/1, Fcn9/1
  BryantISO [deg]/1 -> xyz 2 zxy/1  "BryantAngles rotx roty rotz Visu"
  RotMat2AxisAngle/1(Angles_Visu) -> zxy 2 xyz/1
  Mux1/1 -> RotMat2AxisAngle/1(RotMat_Visu)  "RotationMatrix Visu"
  Fcn17/1 -> Mux1/9
  Fcn16/1 -> Mux1/8
  Fcn15/1 -> Mux1/7
  Fcn14/1 -> Mux1/6
  Fcn13/1 -> Mux1/5
  Fcn12/1 -> Mux1/4
  Fcn11/1 -> Mux1/3
  Fcn10/1 -> Mux1/2
  Fcn9/1 -> Mux1/1
